simulink library "pathFollowingController_cl"  (R2018b)
settings: Solver=VariableStepAuto  StartTime=0.0  StopTime=10.0  RelTol=1e-3
undefined symbols (not defined in the file): max_bank
libraries: filteredPIDController_ul x4, eulAng2RotMat_ul x1, schmehlTangentRotation_ul x1
settings Model: Creator=jldanie5  LastModifiedBy=jldanie5

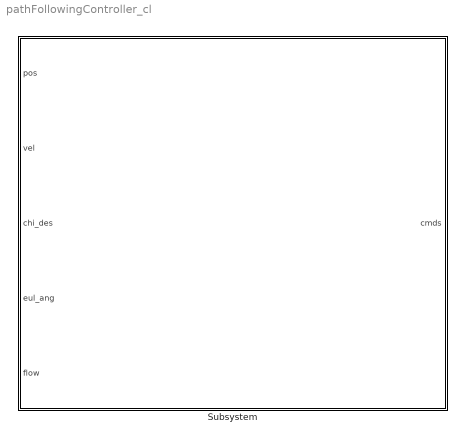
== system pathFollowingController_cl ==
  Subsystem : Subsystem  mask{AoA_des=0, controlMat=0, ctrlSigMax=0}
      mask prompts: AoA_des "Desired Angle of Attack"; controlMat "Matrix to convert Desired Moments to Control Signals"; ctrlSigMax "Max control signal"

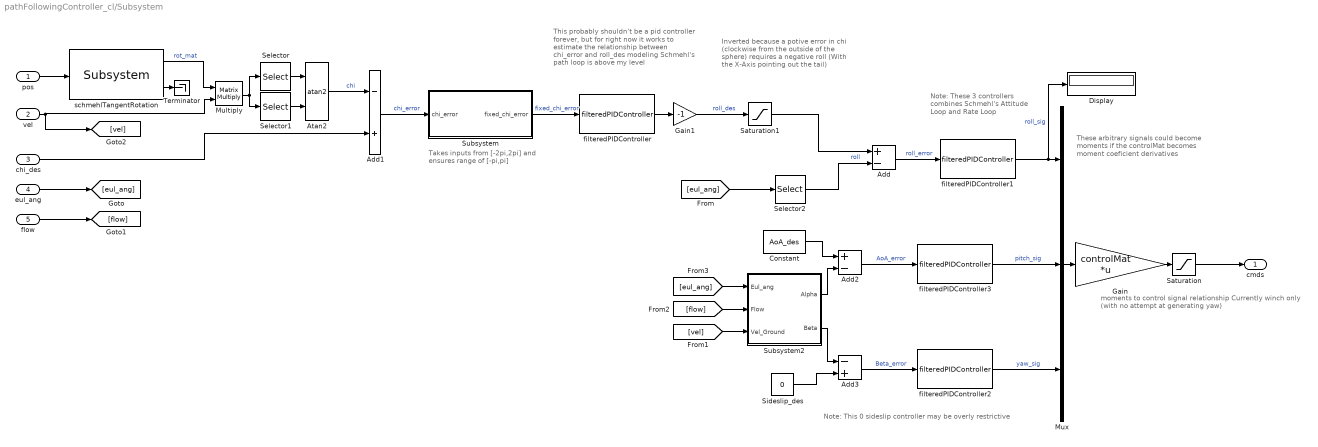
== system pathFollowingController_cl/Subsystem ==
  note: These arbitrary signals could become
      | moments if the controlMat
      | becomes moment coeficient derivatives
  note: Inverted because a potive error
      | in chi (clockwise from the outside of
      | the sphere) requires a negative roll
      | (With the X-Axis pointing out the tail)
  note: Note: These 3 controllers
      | combines Schmehl's Attitude
      | Loop and Rate Loop
  note: Note: This 0 sideslip controller may be overly restrictive
  note: This probably shouldn't be a pid
      | controller forever, but for right now
      | it works to estimate the relationship
      | between chi_error and roll_des
      |
      | modeling Schmehl's path loop is above
      | my level
  note: Takes inputs from [-2pi,2pi] and
      | ensures range of [-pi,pi]
  note: moments to control signal relationship
      | Currently winch only (with no attempt at generating yaw)
  pos : Inport
  vel : Inport  Port=2
  chi_des : Inport  Port=3
  eul_ang : Inport  Port=4
  flow : Inport  Port=5
  Add : Sum  Inputs=+-
  Add1 : Sum  Inputs=-+
  Add2 : Sum  Inputs=+-
  Add3 : Sum  Inputs=-+
  Atan2 : Trigonometry  Operator=atan2
  Constant : Constant  Value=AoA_des
  Display : Display
  Gain : Gain  Gain=controlMat  Multiplication=Matrix(K*u)
  Gain1 : Gain  Gain=-1
  Multiply : Product  Multiplication=Matrix(*)
  Mux : Mux  Inputs=3
  Saturation : Saturate  UpperLimit=ctrlSigMax  LowerLimit=-ctrlSigMax
  Saturation1 : Saturate  UpperLimit=max_bank  LowerLimit=-max_bank
  Selector : Selector  InputPortWidth=3  IndexOptions=Index vector (dialog)  Indices=2  OutputSizes=1
  Selector1 : Selector  InputPortWidth=3  IndexOptions=Index vector (dialog)  Indices=1  OutputSizes=1
  Selector2 : Selector  InputPortWidth=3  IndexOptions=Index vector (dialog)  Indices=1  OutputSizes=1
  Sideslip_des : Constant  Value=0
  Subsystem : Subsystem
  Subsystem2 : Subsystem
  Terminator : Terminator
  filteredPIDController : filteredPIDController_ul/filteredPIDController  kp=kp_chi  ki=0  kd=kd_chi  tau=tau_chi
  filteredPIDController1 : filteredPIDController_ul/filteredPIDController  kp=kp_L  ki=0  kd=kd_L  tau=tau_L
  filteredPIDController2 : filteredPIDController_ul/filteredPIDController  kp=kp_L  ki=0  kd=kd_L  tau=tau_L
  filteredPIDController3 : filteredPIDController_ul/filteredPIDController  kp=kp_M  ki=0  kd=kd_M  tau=tau_M
  schmehlTangentRotation : schmehlTangentRotation_ul/Subsystem  SystemSampleTime=-1
  cmds : Outport
  wires:
  schmehlTangentRotation/2 -> Terminator/1
  schmehlTangentRotation/1 -> Multiply/1  "rot_mat"
  pos/1 -> schmehlTangentRotation/1
  vel/1 -> Multiply/2, [vel]
  Multiply/1 -> Selector/1, Selector1/1
  Selector1/1 -> Atan2/2
  Selector/1 -> Atan2/1
  Atan2/1 -> Add1/1  "chi"
  chi_des/1 -> Add1/2
  [eul_ang] -> Selector2/1
  Selector2/1 -> Add/2  "roll"
  Add/1 -> filteredPIDController1/1  "roll_error"
  filteredPIDController1/1 -> Display/1, Mux/1  "roll_sig"
  Mux/1 -> Gain/1
  eul_ang/1 -> [eul_ang]
  flow/1 -> [flow]
  Add1/1 -> Subsystem/1(chi_error)  "chi_error"
  Subsystem/1(fixed_chi_error) -> filteredPIDController/1  "fixed_chi_error"
  filteredPIDController/1 -> Gain1/1
  filteredPIDController2/1 -> Mux/3  "yaw_sig"
  filteredPIDController3/1 -> Mux/2  "pitch_sig"
  [eul_ang] -> Subsystem2/1(Eul_ang)
  [flow] -> Subsystem2/2(Flow)
  [vel] -> Subsystem2/3(Vel_Ground)
  Subsystem2/1(Alpha) -> Add2/2
  Constant/1 -> Add2/1
  Add2/1 -> filteredPIDController3/1  "AoA_error"
  Subsystem2/2(Beta) -> Add3/1
  Sideslip_des/1 -> Add3/2
  Add3/1 -> filteredPIDController2/1  "Beta_error"
  Gain/1 -> Saturation/1
  Saturation/1 -> cmds/1
  Gain1/1 -> Saturation1/1  "roll_des"
  Saturation1/1 -> Add/1

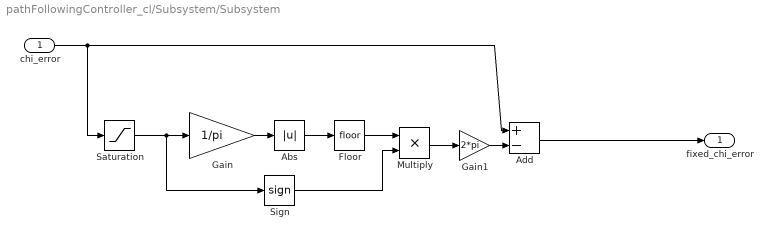
== system pathFollowingController_cl/Subsystem/Subsystem ==
  chi_error : Inport
  Abs : Abs
  Add : Sum  Inputs=+-
  Floor : Rounding
  Gain : Gain  Gain=1/pi
  Gain1 : Gain  Gain=2*pi
  Multiply : Product
  Saturation : Saturate  UpperLimit=pi  LowerLimit=-pi
  Sign : Signum
  fixed_chi_error : Outport
  wires:
  Add/1 -> fixed_chi_error/1
  chi_error/1 -> Saturation/1, Add/1
  Saturation/1 -> Sign/1, Gain/1
  Gain/1 -> Abs/1
  Abs/1 -> Floor/1
  Floor/1 -> Multiply/1
  Sign/1 -> Multiply/2
  Multiply/1 -> Gain1/1
  Gain1/1 -> Add/2

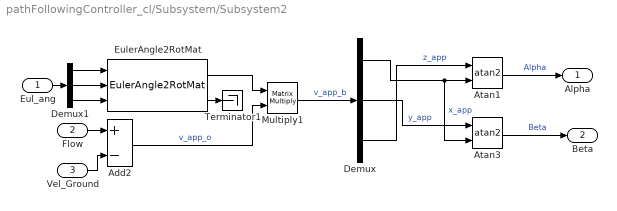
== system pathFollowingController_cl/Subsystem/Subsystem2 ==
  Eul_ang : Inport
  Flow : Inport  Port=2
  Vel_Ground : Inport  Port=3
  Add2 : Sum  Inputs=+-
  Atan1 : Trigonometry  Operator=atan2
  Atan3 : Trigonometry  Operator=atan2
  Demux : Demux  Outputs=3
  Demux1 : Demux  Outputs=3
  EulerAngle2RotMat : eulAng2RotMat_ul/EulerAngle2RotMat  SystemSampleTime=-1
  Multiply1 : Product  Multiplication=Matrix(*)
  Terminator1 : Terminator
  Alpha : Outport
  Beta : Outport  Port=2
  wires:
  Demux/1 -> Atan1/2, Atan3/2  "x_app"
  EulerAngle2RotMat/2 -> Terminator1/1
  Demux/3 -> Atan1/1  "z_app"
  Demux/2 -> Atan3/1  "y_app"
  EulerAngle2RotMat/1 -> Multiply1/1
  Multiply1/1 -> Demux/1  "v_app_b"
  Eul_ang/1 -> Demux1/1
  Add2/1 -> Multiply1/2  "v_app_o"
  Atan3/1 -> Beta/1  "Beta"
  Flow/1 -> Add2/1
  Atan1/1 -> Alpha/1  "Alpha"
  Vel_Ground/1 -> Add2/2
  Demux1/3 -> EulerAngle2RotMat/3
  Demux1/2 -> EulerAngle2RotMat/2
  Demux1/1 -> EulerAngle2RotMat/1
